simulink model "virtual_parent"  (R2016b)
settings: Solver=FixedStepDiscrete  StartTime=0.0  StopTime=10.0  FixedStep=0.2  RelTol=1e-3
values from neighbouring files (symbols this model uses):
  param_A = Simulink.Parameter    [virtual_parent_init.m]
  param_B = Simulink.Parameter    [virtual_parent_init.m]
settings Model: Creator=developer  LastModifiedBy=developer
settings OptimizationCC: BlockReduction=off  DefaultParameterBehavior=Inlined  UseDivisionForNetSlopeComputation=on  ExpressionFolding=off  PassReuseOutputArgsAs=Individual arguments
settings DebuggingCC: ParameterTunabilityLossMsg=error  AssertControl=DisableAll
settings RTWCC: SystemTargetFile=ert.tlc  TemplateMakefile=ert_default_tmf  Description=Embedded Coder
settings CodeAppCC: ForceParamTrailComments=on  IgnoreCustomStorageClasses=off  OperatorAnnotations=on  SimulinkDataObjDesc=on  SFDataObjDesc=on  MATLABFcnDesc=on  InsertBlockDesc=on  MATLABSourceComments=on  EnableCustomComments=on  InlinedPrmAccess=Macros  ReqsInCode=on
settings ERTTargetCC: TargetLangStandard=C99 (ISO)  UtilityFuncGeneration=Shared location  MultiwordLength=256  GenerateSampleERTMain=on  SupportNonFinite=off  ParenthesesLevel=Maximum  CastingMode=Standards  InlinedParameterPlacement=NonHierarchical  ERTCustomFileTemplate=example_file_process.tlc  ConvertIfToSwitch=off  EnableSignedLeftShifts=off  EnableSignedRightShifts=off

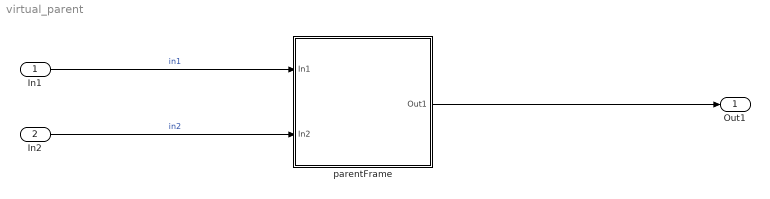
== system virtual_parent ==
  In1 : Inport
  In2 : Inport  Port=2
  parentFrame : Subsystem
  Out1 : Outport
  wires:
  In1/1 -> parentFrame/1(In1)  "in1"
  In2/1 -> parentFrame/2(In2)  "in2"
  parentFrame/1(Out1) -> Out1/1

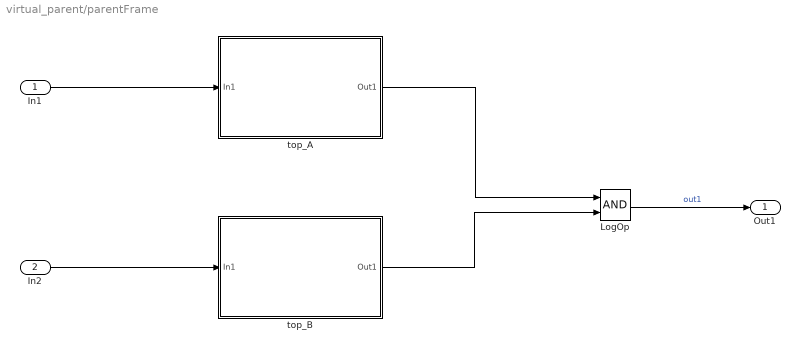
== system virtual_parent/parentFrame ==
  In1 : Inport
  In2 : Inport  Port=2
  LogOp : Logic  AllPortsSameDT=off  OutDataTypeStr=boolean
  top_A : Subsystem  TreatAsAtomicUnit=on  RTWFcnName=func_A
      settings: RTWSystemCode=Nonreusable function  RTWFcnNameOpts=User specified
  top_B : Subsystem  TreatAsAtomicUnit=on  RTWFcnName=func_B
      settings: RTWSystemCode=Nonreusable function  RTWFcnNameOpts=User specified
  Out1 : Outport
  wires:
  top_B/1(Out1) -> LogOp/2
  In2/1 -> top_B/1(In1)
  top_A/1(Out1) -> LogOp/1
  LogOp/1 -> Out1/1  "out1"
  In1/1 -> top_A/1(In1)

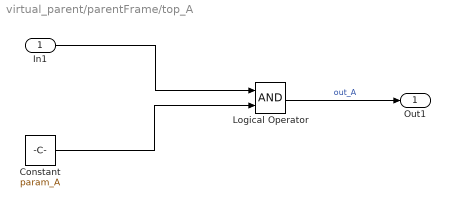
== system virtual_parent/parentFrame/top_A ==
  In1 : Inport
  Constant : Constant  Value=param_A
  Logical Operator : Logic  AllPortsSameDT=off  OutDataTypeStr=boolean
  Out1 : Outport
  wires:
  Logical Operator/1 -> Out1/1  "out_A"
  Constant/1 -> Logical Operator/2
  In1/1 -> Logical Operator/1

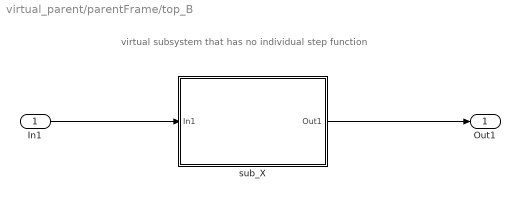
== system virtual_parent/parentFrame/top_B ==
  note: virtual subsystem that has no individual step function
  In1 : Inport
  sub_X : Subsystem
  Out1 : Outport
  wires:
  In1/1 -> sub_X/1(In1)
  sub_X/1(Out1) -> Out1/1

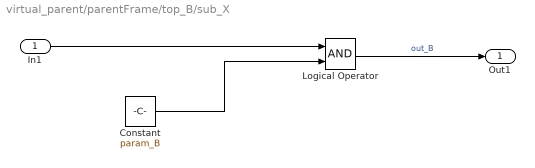
== system virtual_parent/parentFrame/top_B/sub_X ==
  In1 : Inport
  Constant : Constant  Value=param_B
  Logical Operator : Logic  AllPortsSameDT=off  OutDataTypeStr=boolean
  Out1 : Outport
  wires:
  Logical Operator/1 -> Out1/1  "out_B"
  Constant/1 -> Logical Operator/2
  In1/1 -> Logical Operator/1
